simulink subsystem "Torque_Control"  (R2026a)
settings: Solver=VariableStepAuto
undefined symbols (not defined in the file): Iq_max, K_t2iq

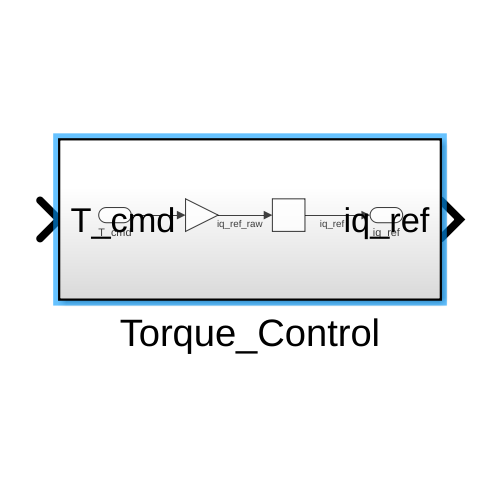
[thumbnail: Simulink's stored preview of the top-level diagram]
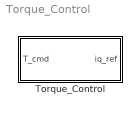
== system Torque_Control ==
  Torque_Control : Subsystem

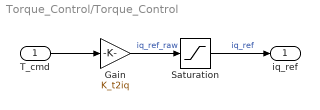
== system Torque_Control/Torque_Control ==
  T_cmd : Inport
  Gain : Gain  Gain=K_t2iq
  Saturation : Saturate  UpperLimit=Iq_max  LowerLimit=-Iq_max
  iq_ref : Outport
  wires:
  T_cmd/1 -> Gain/1
  Gain/1 -> Saturation/1  "iq_ref_raw"
  Saturation/1 -> iq_ref/1  "iq_ref"
